simulink model "MPC_Design_2_R2022b"  (R2022b)
settings: Solver=ode5  StartTime=0  StopTime=7  FixedStep=Ts  RelTol=1e-3
InitFcn:
  | Init_Model;
StartFcn:
  | Init_Model;
values from neighbouring files (symbols this model uses):
  p = data.PredictionHorizon    [CostFunctionAerationJacobian.m]    (also in MPC_Design_V2.m = 10)
  ref = data.References(2)    [CostFunctionAerationJacobian.m]    (also in MPC_Design_V2.m = [(0 - Norm.C(3))/Norm.S(3),     (4 - Norm.C(4))/Norm.S(4)])
  Ts = 15/(24*60)    (= 0.0104166666667)    [MPC_Design_V2.m]
undefined symbols (not defined in the file or in its folder): DOMAX, Norm, OO
libraries: slident x1, mpclib x1
settings Model: Creator=Selim  LastModifiedBy=Selim
settings OptimizationCC: ReuseModelBlockBuffer=on

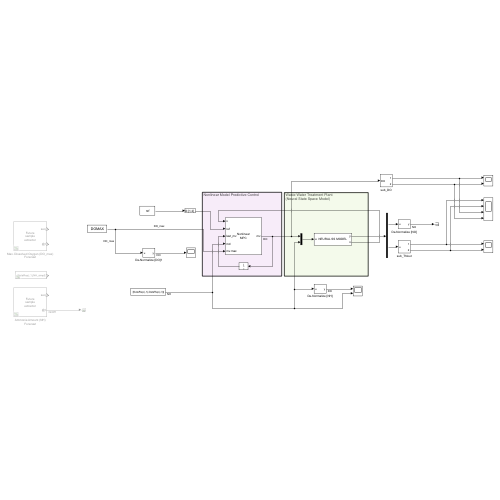
[thumbnail: Simulink's stored preview of the top-level diagram]
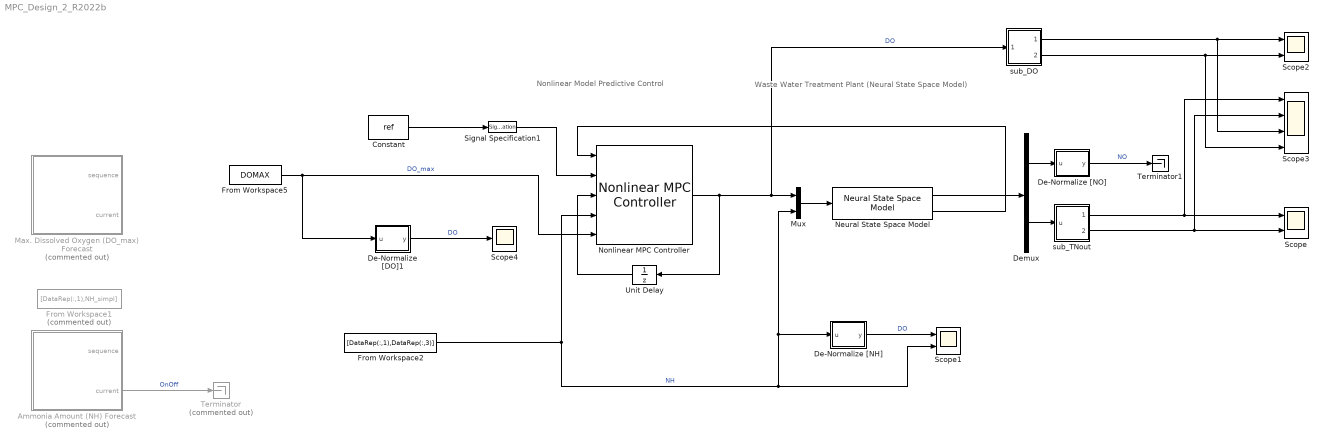
== system MPC_Design_2_R2022b ==
  note: Waste Water Treatment Plant
      | (Neural State Space Model)
  note: Nonlinear Model Predictive Control
  Ammonia Amount (NH) Forecast : Subsystem  Commented=on  mask{signal=OO, ts=Ts, steps=p}
      mask prompts: signal "Signal name"; ts "Sampling time"; steps "Number of previewing steps"
      mask init:
      | ts = evalin('base',get_param(gcbh,'ts'));
      | signal = evalin('base',get_param(gcbh,'signal'));
      | steps = evalin('base',get_param(gcbh,'steps'));
      | data = mpc_previewer_maskinit(signal,ts);
      mask Display:
      | fprintf('Future\nsample\nextractor');
      | port_label('output', 1, 'seq')
      | port_label('output', 2, '@t')
  Constant : Constant  Value=ref
  De-Normalize [DO]1 : Subsystem
  De-Normalize [NH] : Subsystem
  De-Normalize [NO] : Subsystem
  Demux : Demux  Outputs=2
  From Workspace1 : FromWorkspace  Commented=on  VariableName=[DataRep(:,1),NH_simpl]
  From Workspace2 : FromWorkspace  VariableName=[DataRep(:,1),DataRep(:,3)]
  From Workspace5 : FromWorkspace  VariableName=DOMAX
  Max. Dissolved Oxygen (DO_max) Forecast : Subsystem  Commented=on  mask{signal=DOMAX, ts=Ts, steps=p-1}
      mask prompts: signal "Signal name"; ts "Sampling time"; steps "Number of previewing steps"
      mask init:
      | ts = evalin('base',get_param(gcbh,'ts'));
      | signal = evalin('base',get_param(gcbh,'signal'));
      | steps = evalin('base',get_param(gcbh,'steps'));
      | data = mpc_previewer_maskinit(signal,ts);
      mask Display:
      | fprintf('Future\nsample\nextractor');
      | port_label('output', 1, 'seq')
      | port_label('output', 2, '@t')
  Mux : Mux  Inputs=2
  Neural State Space Model : slident/Models/Neural State Space Model  sys=sys  x0type=internal  ic=x0  returnx=on  returndx=off  domain=CT  feedthroughCT=NoFT  feedthroughDT=FT
  Nonlinear MPC Controller : mpclib/Nonlinear MPC Controller  nlmpcobj=nlobj  UseObjectTs=on  UseMEX=off  md_enabled=on  mvtarget_enabled=off  param_enabled=off  cost_enabled=off  mvseq_enabled=off  stateseq_enabled=off  ovseq_enabled=off  slack_enabled=off  status_enabled=off  ov_min=off  ov_max=off  mv_min=off  mv_max=on  mvrate_min=off  mvrate_max=off  state_min=off  state_max=off  ov_weight=off  mv_weight=off  mvrate_weight=off  ecr_weight=off  nlp_initialize=off
  Scope : Scope  NumInputPorts=2
  Scope1 : Scope  NumInputPorts=2
  Scope2 : Scope  NumInputPorts=2
  Scope3 : Scope  NumInputPorts=4
  Scope4 : Scope
  Signal Specification1 : SignalSpecification  Dimensions=[1,2]
  Terminator : Terminator  Commented=on
  Terminator1 : Terminator
  Unit Delay : UnitDelay  SampleTime=-1  HasFrameUpgradeWarning=on
  sub_DO : Subsystem
  sub_TNout : Subsystem
  wires:
  Unit Delay/1 -> Nonlinear MPC Controller/3
  Mux/1 -> Neural State Space Model/1
  Demux/1 -> De-Normalize [NO]/1(u)
  De-Normalize [NO]/1(y) -> Terminator1/1  "NO"
  Neural State Space Model/1 -> Demux/1
  Constant/1 -> Signal Specification1/1
  Signal Specification1/1 -> Nonlinear MPC Controller/2
  From Workspace2/1 -> Scope1/2, De-Normalize [NH]/1(u), Mux/2, Nonlinear MPC Controller/4  "NH"
  Ammonia Amount (NH) Forecast/2(current) -> Terminator/1  "OnOff"
  Nonlinear MPC Controller/1 -> sub_DO/1(DO), Mux/1, Unit Delay/1  "DO"
  From Workspace5/1 -> De-Normalize [DO]1/1(u), Nonlinear MPC Controller/5  "DO_max"
  De-Normalize [NH]/1(y) -> Scope1/1  "DO"
  Neural State Space Model/2 -> Nonlinear MPC Controller/1
  De-Normalize [DO]1/1(y) -> Scope4/1  "DO"
  Demux/2 -> sub_TNout/1(u)
  sub_TNout/1(Out1) -> Scope3/1, Scope/1
  sub_TNout/2(Out2) -> Scope3/2, Scope/2
  sub_DO/1(Out1) -> Scope3/3, Scope2/1
  sub_DO/2(Out2) -> Scope3/4, Scope2/2

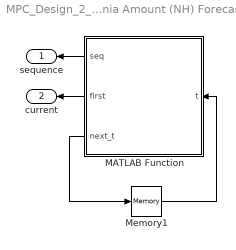
== system MPC_Design_2_R2022b/Ammonia Amount (NH) Forecast ==
  MATLAB Function : MATLAB Function  TreatAsAtomicUnit=on
  Memory1 : Memory  InheritSampleTime=on  LinearizeAsDelay=on
  sequence : Outport  VectorParamsAs1DForOutWhenUnconnected=off
  current : Outport  Port=2  VectorParamsAs1DForOutWhenUnconnected=off
  wires:
  MATLAB Function/3(next_t) -> Memory1/1
  Memory1/1 -> MATLAB Function/1(t)
  MATLAB Function/2(first) -> current/1
  MATLAB Function/1(seq) -> sequence/1

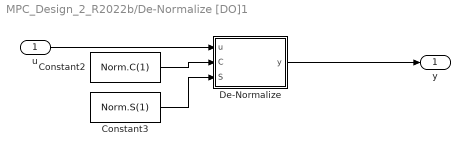
== system MPC_Design_2_R2022b/De-Normalize [DO]1 ==
  u : Inport
  Constant2 : Constant  Value=Norm.C(1)
  Constant3 : Constant  Value=Norm.S(1)
  De-Normalize : MATLAB Function  TreatAsAtomicUnit=on
  y : Outport
  wires:
  Constant3/1 -> De-Normalize/3(S)
  u/1 -> De-Normalize/1(u)
  De-Normalize/1(y) -> y/1
  Constant2/1 -> De-Normalize/2(C)

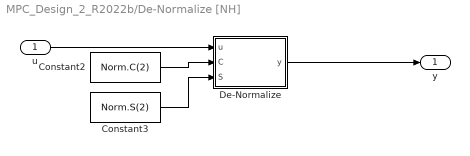
== system MPC_Design_2_R2022b/De-Normalize [NH] ==
  u : Inport
  Constant2 : Constant  Value=Norm.C(2)
  Constant3 : Constant  Value=Norm.S(2)
  De-Normalize : MATLAB Function  TreatAsAtomicUnit=on
  y : Outport
  wires:
  Constant3/1 -> De-Normalize/3(S)
  u/1 -> De-Normalize/1(u)
  De-Normalize/1(y) -> y/1
  Constant2/1 -> De-Normalize/2(C)

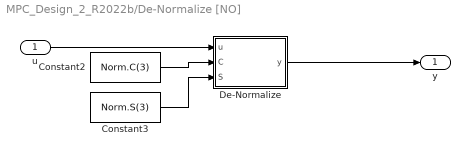
== system MPC_Design_2_R2022b/De-Normalize [NO] ==
  u : Inport
  Constant2 : Constant  Value=Norm.C(3)
  Constant3 : Constant  Value=Norm.S(3)
  De-Normalize : MATLAB Function  TreatAsAtomicUnit=on
  y : Outport
  wires:
  Constant3/1 -> De-Normalize/3(S)
  u/1 -> De-Normalize/1(u)
  De-Normalize/1(y) -> y/1
  Constant2/1 -> De-Normalize/2(C)

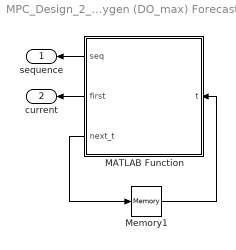
== system MPC_Design_2_R2022b/Max. Dissolved Oxygen (DO_max) Forecast ==
  MATLAB Function : MATLAB Function  TreatAsAtomicUnit=on
  Memory1 : Memory  InheritSampleTime=on  LinearizeAsDelay=on
  sequence : Outport  VectorParamsAs1DForOutWhenUnconnected=off
  current : Outport  Port=2  VectorParamsAs1DForOutWhenUnconnected=off
  wires:
  MATLAB Function/1(seq) -> sequence/1
  MATLAB Function/2(first) -> current/1
  Memory1/1 -> MATLAB Function/1(t)
  MATLAB Function/3(next_t) -> Memory1/1

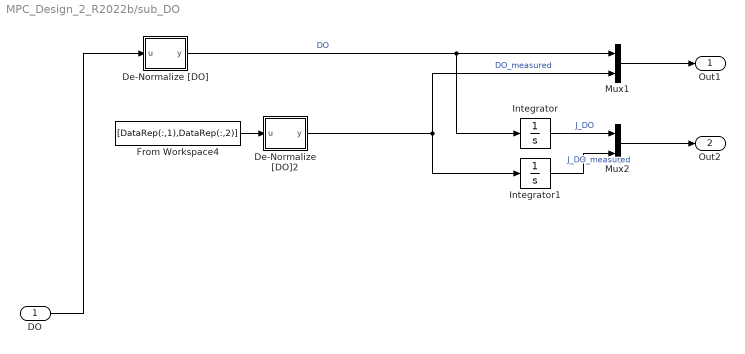
== system MPC_Design_2_R2022b/sub_DO ==
  DO : Inport
  De-Normalize [DO] : Subsystem
  De-Normalize [DO]2 : Subsystem
  From Workspace4 : FromWorkspace  VariableName=[DataRep(:,1),DataRep(:,2)]
  Integrator : Integrator
  Integrator1 : Integrator
  Mux1 : Mux  Inputs=2
  Mux2 : Mux  Inputs=2
  Out1 : Outport
  Out2 : Outport  Port=2
  wires:
  Integrator1/1 -> Mux2/2  "J_DO_measured"
  Integrator/1 -> Mux2/1  "J_DO"
  De-Normalize [DO]/1(y) -> Mux1/1, Integrator/1  "DO"
  DO/1 -> De-Normalize [DO]/1(u)
  From Workspace4/1 -> De-Normalize [DO]2/1(u)
  Mux2/1 -> Out2/1
  De-Normalize [DO]2/1(y) -> Integrator1/1, Mux1/2  "DO_measured"
  Mux1/1 -> Out1/1

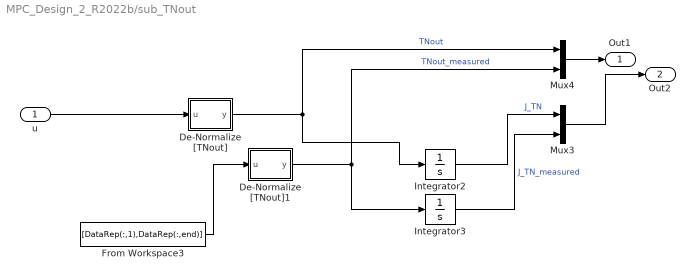
== system MPC_Design_2_R2022b/sub_TNout ==
  u : Inport
  De-Normalize [TNout] : Subsystem
  De-Normalize [TNout]1 : Subsystem
  From Workspace3 : FromWorkspace  VariableName=[DataRep(:,1),DataRep(:,end)]
  Integrator2 : Integrator
  Integrator3 : Integrator
  Mux3 : Mux  Inputs=2
  Mux4 : Mux  Inputs=2
  Out1 : Outport
  Out2 : Outport  Port=2
  wires:
  De-Normalize [TNout]1/1(y) -> Mux4/2, Integrator3/1  "TNout_measured"
  Integrator3/1 -> Mux3/2  "J_TN_measured"
  De-Normalize [TNout]/1(y) -> Mux4/1, Integrator2/1  "TNout"
  Mux3/1 -> Out2/1
  u/1 -> De-Normalize [TNout]/1(u)
  Integrator2/1 -> Mux3/1  "J_TN"
  From Workspace3/1 -> De-Normalize [TNout]1/1(u)
  Mux4/1 -> Out1/1

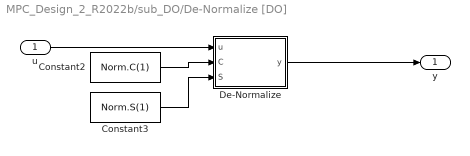
== system MPC_Design_2_R2022b/sub_DO/De-Normalize [DO] ==
  u : Inport
  Constant2 : Constant  Value=Norm.C(1)
  Constant3 : Constant  Value=Norm.S(1)
  De-Normalize : MATLAB Function  TreatAsAtomicUnit=on
  y : Outport
  wires:
  Constant2/1 -> De-Normalize/2(C)
  De-Normalize/1(y) -> y/1
  u/1 -> De-Normalize/1(u)
  Constant3/1 -> De-Normalize/3(S)

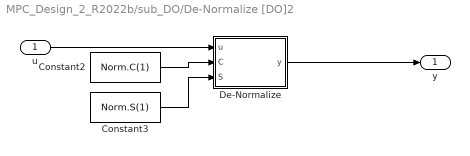
== system MPC_Design_2_R2022b/sub_DO/De-Normalize [DO]2 ==
  u : Inport
  Constant2 : Constant  Value=Norm.C(1)
  Constant3 : Constant  Value=Norm.S(1)
  De-Normalize : MATLAB Function  TreatAsAtomicUnit=on
  y : Outport
  wires:
  Constant3/1 -> De-Normalize/3(S)
  u/1 -> De-Normalize/1(u)
  De-Normalize/1(y) -> y/1
  Constant2/1 -> De-Normalize/2(C)

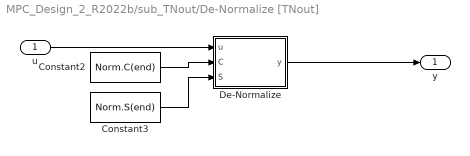
== system MPC_Design_2_R2022b/sub_TNout/De-Normalize [TNout] ==
  u : Inport
  Constant2 : Constant  Value=Norm.C(end)
  Constant3 : Constant  Value=Norm.S(end)
  De-Normalize : MATLAB Function  TreatAsAtomicUnit=on
  y : Outport
  wires:
  Constant2/1 -> De-Normalize/2(C)
  De-Normalize/1(y) -> y/1
  u/1 -> De-Normalize/1(u)
  Constant3/1 -> De-Normalize/3(S)

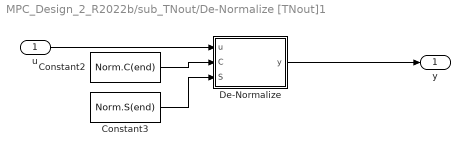
== system MPC_Design_2_R2022b/sub_TNout/De-Normalize [TNout]1 ==
  u : Inport
  Constant2 : Constant  Value=Norm.C(end)
  Constant3 : Constant  Value=Norm.S(end)
  De-Normalize : MATLAB Function  TreatAsAtomicUnit=on
  y : Outport
  wires:
  Constant3/1 -> De-Normalize/3(S)
  u/1 -> De-Normalize/1(u)
  De-Normalize/1(y) -> y/1
  Constant2/1 -> De-Normalize/2(C)

== matlab function MPC_Design_2_R2022b/De-Normalize [NO]/De-Normalize ==
  data: u input; y output; C input; S input
function y = fcn(u,C,S)

y = u * S + C;

end

== matlab function MPC_Design_2_R2022b/sub_DO/De-Normalize [DO]/De-Normalize ==
  data: u input; y output; C input; S input
function y = fcn(u,C,S)

y = u * S + C;

end

== matlab function MPC_Design_2_R2022b/sub_TNout/De-Normalize [TNout]/De-Normalize ==
  data: u input; y output; C input; S input
function y = fcn(u,C,S)

y = u * S + C;

end

== matlab function MPC_Design_2_R2022b/Max. Dissolved Oxygen (DO_max) Forecast/MATLAB Function ==
  settings: updateMethod=DISCRETE  sampleTime=ts
  data: data parameter; seq output; steps parameter; t input; first output; next_t output
function [seq,first,next_t] = fcn(data,steps,t)
%#codegen
[seq,first,next_t] = mpcblock_preview('md',data,steps,t);

== matlab function MPC_Design_2_R2022b/Ammonia Amount (NH) Forecast/MATLAB Function ==
  settings: updateMethod=DISCRETE  sampleTime=ts
  data: data parameter; seq output; steps parameter; t input; first output; next_t output
function [seq,first,next_t] = fcn(data,steps,t)
%#codegen
[seq,first,next_t] = mpcblock_preview('md',data,steps,t);

== matlab function MPC_Design_2_R2022b/De-Normalize [NH]/De-Normalize ==
  data: u input; y output; C input; S input
function y = fcn(u,C,S)

y = u * S + C;

end

== matlab function MPC_Design_2_R2022b/De-Normalize [DO]1/De-Normalize ==
  data: u input; y output; C input; S input
function y = fcn(u,C,S)

y = u * S + C;

end

== matlab function MPC_Design_2_R2022b/sub_TNout/De-Normalize [TNout]1/De-Normalize ==
  data: u input; y output; C input; S input
function y = fcn(u,C,S)

y = u * S + C;

end

== matlab function MPC_Design_2_R2022b/sub_DO/De-Normalize [DO]2/De-Normalize ==
  data: u input; y output; C input; S input
function y = fcn(u,C,S)

y = u * S + C;

end
